simulink model "P5"  (R2022a)
settings: Solver=VariableStepAuto  StartTime=0.0  StopTime=10.0  RelTol=1e-3
undefined symbols (not defined in the file): A, B, C, D, IC
settings Model: Creator=Richi  LastModifiedBy=Richi

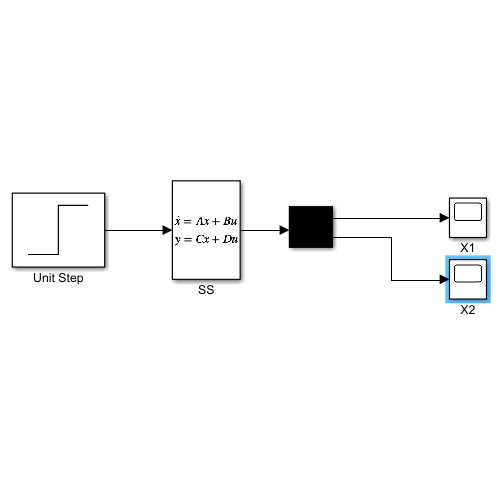
[thumbnail: Simulink's stored preview of the top-level diagram]
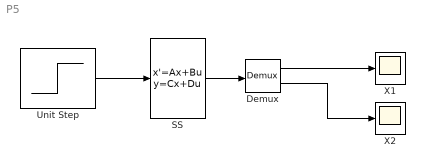
== system P5 ==
  Demux : Demux  Outputs=2
  SS : StateSpace  A=A  B=B  C=C  D=D  InitialCondition=IC
  Unit Step : Step  Time=0  SampleTime=0
  X1 : Scope
  X2 : Scope
  wires:
  Demux/2 -> X2/1
  Demux/1 -> X1/1
  SS/1 -> Demux/1
  Unit Step/1 -> SS/1
